simulink library "sm_solar_tracker_lib"  (R2021b)
settings: Solver=VariableStepAuto  StartTime=0.0  StopTime=10.0  RelTol=1e-3
undefined symbols (not defined in the file or in its folder): X, Y, Z
libraries: sm_lib x89, $bdroot x18
(part 1 of 3)
Description:
  | Solar Tracker Library
settings Model: Creator=The MathWorks, Inc.  LastModifiedBy=The MathWorks, Inc.
settings SolverCC: AlgebraicLoopSolver=TrustRegion
settings DataIOCC: ReturnWorkspaceOutputs=off
settings DebuggingCC: SFMachineParentedDataDiag=warning  ArithmeticOperatorsInVariantConditions=warning
settings SFSimCC: SimUseLocalCustomCode=off  CustomCodeUndefinedFunction=UseInterfaceOnly
settings RTWCC: RTWUseLocalCustomCode=off
settings CodeAppCC: StateflowObjectComments=on
settings ConfigComp: CovMetricSettings=dswe

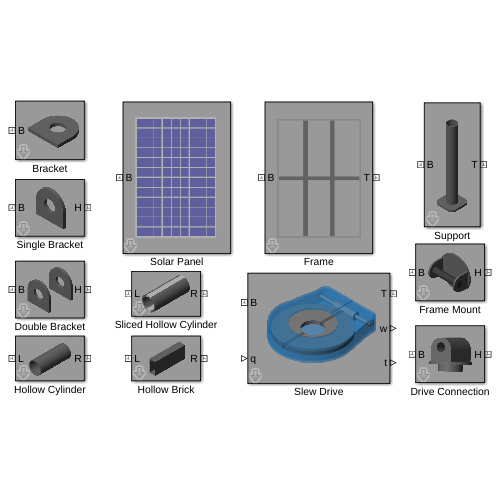
[thumbnail: Simulink's stored preview of the top-level diagram]
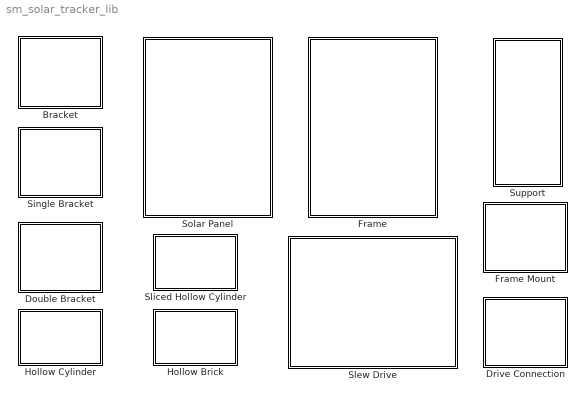
== system sm_solar_tracker_lib ==
  Bracket : Subsystem  mask(Bracket){height=0.1, width=0.1, thickness=0.01, holeOffset=0.05, holeRadius=0.02, rho=2700, color=[0.5 0.5 0.5]}
      mask prompts: height "Height (m)"; width "Width (m)"; thickness "Thickness (m)"; holeOffset "Hole Offset (m)"; holeRadius "Hole Radius (m)"; rho "Density (kg/m^3)"; color "Color [r g b]"
      mask help:
      | This block models a bracket element.
      |
      | Port B corresponds to the center point of the base face.
      mask init:
      | points = 40;
      | 
      | y = height - 0.5*width;
      | 
      | outerVertices = ...
      |   [          0      0;...
      |      0.5*width      0;...
      |      0.5*width      y;...
      |      0.5*width height;...
      |     -0.5*width height;...
      |     -0.5*width      y;...
      |     -0.5*width      0;...
      |              0      0];
      | 
      | outer = simmechanics.demohelpers.round_corners(...
      |   outerVertices, [4 5], 0.5*width, points);
      | 
      | holeTheta = linspace(1.5*pi, -0.5*pi, points);
      | 
      | hole = [holeRadius*cos(holeTheta);...
      |         holeRadius*sin(holeTheta)+holeOffset]';
      | 
      | crossSection = [hole; outer];
      mask DialogControl Tab1 Prompt: Dimensions
      mask DialogControl Tab2 Prompt: Material Properties
      mask Display:
      | image(fullfile(matlabroot,'toolbox','physmod','sm','smdemos','solar_tracker','images','sm_solar_tracker_bracket.png'));
      | port_label('lconn',1,'B');
  Double Bracket : Subsystem  mask(Double Bracket){height=0.75, width=0.75, thickness=0.15, offset=0.8, holeOffset=0.5, holeRadius=0.075, rho=7800, color=[0.3 0.3 0.3]}
      mask prompts: height "Height (m)"; width "Width (m)"; thickness "Thickness (m)"; offset "Offset (m)"; holeOffset "Hole Offset (m)"; holeRadius "Hole Radius (m)"; rho "Density (kg/m^3)"; color "Color [r g b]"
      mask help:
      | This block models a double bracket element.
      |
      | Port B corresponds to the midpoint between the base faces of the two elements. Port H corresponds to the midpoint between the two holes.
      mask DialogControl Tab1 Prompt: Dimensions
      mask DialogControl Tab2 Prompt: Material Properties
      mask Display:
      | image(fullfile(matlabroot,'toolbox','physmod','sm','smdemos','solar_tracker','images','sm_solar_tracker_double_bracket.png'));
      | port_label('lconn',1,'B');
      | port_label('rconn',1,'H');
  Drive Connection : Subsystem  mask(Drive Connection){connRadius=0.05, connThickness=0.005, connLength=0.03, bracketWidth=0.1, bracketThickness=0.15, holeRadius=0.02, holeOffset=0.06, baseThickness=0.01, rho=2700, color=[0.5 0.5 0.5]}
      mask prompts: connRadius "Connection Radius (m)"; connThickness "Connection Thickness (m)"; connLength "Connection Length (m)"; bracketWidth "Bracket Width and Height (m)"; bracketThickness "Bracket Thickness (m)"; holeRadius "Hole Radius (m)"; holeOffset "Hole Offset (m)"; baseThickness "Base Thickness (m)"; rho "Density (kg/m^3)"; color "Color [r g b]"
      mask help:
      | This block models the element that connects the solar array assembly to the slew drive.
      |
      | Port B corresponds to the center of the base face of the drive connection. Port H corresponds to the center of the bracket hole.
      mask init:
      | baseAngle = atan(bracketWidth / bracketThickness);
      | baseRadius = 0.5 * bracketThickness / cos(baseAngle);
      mask DialogControl Tab1 Prompt: Dimensions
      mask DialogControl Tab2 Prompt: Material Properties
      mask Display:
      | image(fullfile(matlabroot,'toolbox','physmod','sm','smdemos','solar_tracker','images','sm_solar_tracker_drive_connection.png'));
      | port_label('lconn',1,'B');
      | port_label('rconn',1,'H');
  Frame : Subsystem  mask(Frame){width=1, height=1.414, depth=0.1, beamWidth=0.05, beamThickness=0.01, frameWidth=0.02, frameThickness=0.005, rho=2700, beamColor=[0.5 0.5 0.5], frameColor=[0.7 0.7 0.7]}
      mask prompts: width "Width (m)"; height "Height (m)"; depth "Depth (m)"; beamWidth "Beam Width (m)"; beamThickness "Beam Thickness (m)"; frameWidth "Frame Width (m)"; frameThickness "Frame Thickness (m)"; rho "Density (kg/m^3)"; beamColor "Beam Color [r g b]"; frameColor "Frame Color [r g b]"
      mask help:
      | This block models the mounting frame of the solar tracker.
      |
      | Port B corresponds to the center of the base face of the horizontal beam. Port T corresponds to the center of the top face of the horizontal beam.
      mask init:
      | horizBeamLength = width - 2*frameWidth;
      | vertBeamLength = height - 2*frameWidth;
      | 
      | vertBeam1_offset = [-0.5*vertBeamLength 0 -(1/3)*horizBeamLength];
      | vertBeam2_offset = [-0.5*vertBeamLength 0 -(2/3)*horizBeamLength];
      | 
      | baseOffset = [0 -0.5*depth 0.5*horizBeamLength];
      | topOffset  = [0  0.5*depth 0.5*horizBeamLength];
      | 
      | leftFrameOffset  = [-0.5*height 0 -0.5*frameWidth];
      | rightFrameOffset = [-0.5*height 0  0.5*frameWidth];
      | 
      | nearFarFrameOffset = 0.5*height-0.5*frameWidth;
      mask DialogControl Tab1 Prompt: Dimensions
      mask DialogControl Tab2 Prompt: Material Properties
      mask Display:
      | image(fullfile(matlabroot,'toolbox','physmod','sm','smdemos','solar_tracker','images','sm_solar_tracker_frame.png'));
      | port_label('lconn',1,'B');
      | port_label('rconn',1,'T');
  Frame Mount : Subsystem  mask(Frame Mount){bracketWidth=0.1, bracketThickness=0.01, bracketOffset=0.18, holeRadius=0.02, holeOffset=0.06, baseThickness=0.01, rho=2700, mountColor=[0.5 0.5 0.5], pinColor=[0.3 0.3 0.3]}
      mask prompts: bracketWidth "Bracket Width and Height (m)"; bracketThickness "Bracket Thickness (m)"; bracketOffset "Bracket Offset (m)"; holeRadius "Hole Radius (m)"; holeOffset "Hole Offset (m)"; baseThickness "Base Thickness (m)"; rho "Density (kg/m^3)"; mountColor "Mount Color [r g b]"; pinColor "Pin Color [r g b]"
      mask help:
      | This block models the mount for the frame of the solar tracker.
      |
      | Port B corresponds to the center of the base plate. Port H corresponds to the center point of the pin that passes through the holes of the bracket.
      mask init:
      | baseAngle = atan(bracketWidth / (bracketOffset + bracketThickness));
      | baseRadius = 0.5*bracketWidth / sin(baseAngle);
      | pinLength = bracketOffset + bracketThickness;
      mask DialogControl Tab1 Prompt: Dimensions
      mask DialogControl Tab2 Prompt: Material Properties
      mask Display:
      | image(fullfile(matlabroot,'toolbox','physmod','sm','smdemos','solar_tracker','images','sm_solar_tracker_frame_mount.png'));
      | port_label('lconn',1,'B');
      | port_label('rconn',1,'H');
  Hollow Brick : Subsystem  mask(Hollow Brick){width=0.1, depth=0.2, length=0.5, thickness=0.01, rho=2700, color=[0.5 0.5 0.5]}
      mask prompts: width "Width (m)"; depth "Depth (m)"; length "Length (m)"; thickness "Thickness (m)"; rho "Density (kg/m^3)"; color "Color [r g b]"
      mask help:
      | This block models a hollow brick element.
      |
      | Port L corresponds to the left-hand end of the brick. Port R corresponds to the right-hand end of the brick.
      mask init:
      | halfWidth = 0.5*width;
      | halfDepth = 0.5*depth;
      | 
      | halfInnerWidth = 0.5*(width - 2*thickness);
      | halfInnerDepth = 0.5*(depth - 2*thickness);
      | 
      | crossSection = [...
      |   -halfInnerWidth -halfInnerDepth;...
      |   -halfInnerWidth  halfInnerDepth;...
      |    halfInnerWidth  halfInnerDepth;...
      |    halfInnerWidth -halfInnerDepth;...
      |   -halfInnerWidth -halfInnerDepth;...
      |   -halfWidth      -halfDepth;...
      |    halfWidth      -halfDepth;...
      |    halfWidth       halfDepth;...
      |   -halfWidth       halfDepth;...
      |   -halfWidth      -halfDepth];
      mask DialogControl Tab1 Prompt: Dimensions
      mask DialogControl Tab2 Prompt: Material Properties
      mask Display:
      | image(fullfile(matlabroot,'toolbox','physmod','sm','smdemos','solar_tracker','images','sm_solar_tracker_hollow_brick.png'));
      | port_label('lconn',1,'L');
      | port_label('rconn',1,'R');
  Hollow Cylinder : Subsystem  mask(Hollow Cylinder){outerRadius=0.1, thickness=0.01, length=0.5, rho=2700, color=[0.5 0.5 0.5]}
      mask prompts: outerRadius "Outer Radius (m)"; thickness "Thickness (m)"; length "Length (m)"; rho "Density (kg/m^3)"; color "Color [r g b]"
      mask help:
      | This block models a hollow cylinder element.
      |
      | Port L corresponds to the left-hand end of the cylinder. Port R corresponds to the right-hand end of the cylinder.
      mask init:
      | innerRadius = outerRadius - thickness;
      | 
      | halfLength = 0.5*length;
      | 
      | crossSection = [...
      |   innerRadius -halfLength;...
      |   outerRadius -halfLength;...
      |   outerRadius  halfLength;...
      |   innerRadius  halfLength];
      mask DialogControl Tab1 Prompt: Dimensions
      mask DialogControl Tab2 Prompt: Material Properties
      mask Display:
      | image(fullfile(matlabroot,'toolbox','physmod','sm','smdemos','solar_tracker','images','sm_solar_tracker_hollow_cylinder.png'));
      | port_label('lconn',1,'L');
      | port_label('rconn',1,'R');
  Single Bracket : Subsystem  mask(Single Bracket){height=0.1, width=0.1, thickness=0.01, holeOffset=0.05, holeRadius=0.02, rho=2700, color=[0.5 0.5 0.5]}
      mask prompts: height "Height (m)"; width "Width (m)"; thickness "Thickness (m)"; holeOffset "Hole Offset (m)"; holeRadius "Hole Radius (m)"; rho "Density (kg/m^3)"; color "Color [r g b]"
      mask help:
      | This block models a bracket element.
      |
      | Port B corresponds to the center point of the base face. Port H corresponds to the center of the hole.
      mask DialogControl Tab1 Prompt: Dimensions
      mask DialogControl Tab2 Prompt: Material Properties
      mask Display:
      | image(fullfile(matlabroot,'toolbox','physmod','sm','smdemos','solar_tracker','images','sm_solar_tracker_single_bracket.png'));
      | port_label('lconn',1,'B');
      | port_label('rconn',1,'H');
  Slew Drive : Subsystem  mask(Slew Drive){wormLeadAngle=10, wormLength=0.17, gearOuterRadius=0.1, gearInnerRadius=0.03, gearExposedRadius=0.06, ratio=50, housingThickness=0.005, bWormRevolute=1e-6, wormRho=7800, gearRho=7800, housingRho=2700, wormColor=[0.7 0.7 0.7], gearColor=[0.6 0.6 0.6], housingColor=[0.1 0.6 1.0], housingOpacity=0.3}
      mask prompts: wormLeadAngle "Worm Lead Angle (deg)"; wormLength "Worm Length (m)"; gearOuterRadius "Gear Outer Radius (m)"; gearInnerRadius "Gear Inner Radius (m)"; gearExposedRadius "Gear Exposed Radius (m)"; ratio "Ratio (Ng / Nw)"; housingThickness "Housing Thickness (m)"; bWormRevolute "Worm Revolute Damping (Nm/(deg/s))"; wormRho "Worm Density (kg/m^3)"; gearRho "Gear Density (kg/m^3)"; housingRho "Housing Density (kg/m3)"; wormColor "Worm Color [r g b]"; gearColor "Gear Color [r g b]"; housingColor "Housing Color [r g b]"; housingOpacity "Housing Opacity"
      mask help:
      | This block models the slew drive of the solar tracker.
      |
      | Port B corresponds to the base face of the housing aligned with the gear axis. Port T corresponds to the center of the top face of the gear.
      |
      | Input port q specifies the motion actuation signal of the gear revolute. Output port w corresponds to the angular velocity of the worm revolute. Output port t corresponds to the automatically computed actuation torque at the worm revolute necessary to achieve the desired motion signal of the gear revolute.
      mask init:
      | % Worm Properties
      | wormRadius            = gearOuterRadius / (ratio * tand(wormLeadAngle));
      | wormNonThreadedRadius = 0.4*wormRadius;
      | 
      | wormThreadedLength    = 0.4*wormLength;
      | wormNonThreadedLength = 0.5*(wormLength - wormThreadedLength);
      | 
      | wormHoleRadius = 0.5*wormNonThreadedRadius;
      | 
      | wormThreadedThickness    = wormRadius - wormHoleRadius;
      | wormNonThreadedThickness = wormNonThreadedRadius - wormHoleRadius;
      | 
      | wormSliceColor      = 0.75*wormColor;
      | wormSliceProportion = 0.25;
      | 
      | % Worm Offsets
      | wormLeftOffset  = [-0.5*wormLength gearOuterRadius+wormRadius 0];
      | wormRightOffset = [ 0.5*wormLength gearOuterRadius+wormRadius 0];
      | 
      | % Gear Properties
      | gearLength         = wormRadius;
      | gearThickness      = gearOuterRadius - gearInnerRadius;
      | gearSliceThickness = 0.1*gearOuterRadius;
      | gearSliceColor     = 0.75*gearColor;
      | 
      | % Housing Dimensions
      | housingRadTol = 0.05*gearOuterRadius;
      | sideDepth     = 2*wormRadius + 2*housingRadTol;
      | 
      | % Housing Base Vertices
      | baseVertex1_x = 0;
      | baseVertex2_x = housingThickness + housingRadTol + 2*wormRadius;
      | baseVertex3_x = baseVertex2_x + gearOuterRadius;
      | baseVertex4_x = baseVertex3_x + gearOuterRadius + housingRadTol + housingThickness;
      | 
      | baseVertex1_y = -0.5*wormLength - housingThickness;
      | baseVertex2_y = baseVertex1_y;
      | baseVertex3_y = -gearOuterRadius - housingRadTol - housingThickness;
      | baseVertex4_y = baseVertex3_y;
      | 
      | baseVertices = [...
      |   baseVertex1_x  baseVertex1_y;...
      |   baseVertex2_x  baseVertex2_y;...
      |   baseVertex3_x  baseVertex3_y;...
      |   baseVertex4_x  baseVertex4_y;...
      |   baseVertex4_x -baseVertex4_y;...
      |   baseVertex3_x -baseVertex3_y;...
      |   baseVertex2_x -baseVertex2_y;...
      |   baseVertex1_x -baseVertex1_y];
      | 
      | baseVertex1_R = 0.5*wormRadius + housingRadTol + housingThickness;
      | baseVertex4_R = gearOuterRadius + housingRadTol + housingThickness;
      | baseVertex5_R = baseVertex4_R;
      | baseVertex8_R = baseVertex1_R;
      | 
      | baseVerticesR = [baseVertex1_R baseVertex4_R baseVertex5_R baseVertex8_R];
      |   
      | baseVertices = simmechanics.demohelpers.round_corners(...
      |   baseVertices, [1 4 5 8], baseVerticesR, 20);
      | 
      | % Housing Side Vertices
      | sideVertices = [...
      |   baseVertex1_x+housingThickness  baseVertex1_y+housingThickness;...
      |   baseVertex2_x                   baseVertex2_y+housingThickness;...
      |   baseVertex3_x                   baseVertex3_y+housingThickness;...
      |   baseVertex4_x-housingThickness  baseVertex4_y+housingThickness;...
      |   baseVertex4_x-housingThickness -baseVertex4_y-housingThickness;...
      |   baseVertex3_x                  -baseVertex3_y-housingThickness;...
      |   baseVertex2_x                  -baseVertex2_y-housingThickness;...
      |   baseVertex1_x+housingThickness -baseVertex1_y-housingThickness];
      | 
      | sideVertex1_R = 0.5*wormRadius + housingRadTol;
      | sideVertex4_R = gearOuterRadius + housingRadTol;
      | sideVertex5_R = sideVertex4_R;
      | sideVertex8_R = sideVertex1_R;
      | 
      | sideVerticesR = [sideVertex1_R sideVertex4_R sideVertex5_R sideVertex8_R];
      | 
      | sideVertices = simmechanics.demohelpers.round_corners(...
      |   sideVertices, [1 4 5 8], sideVerticesR, 20);
      | 
      | sideVertices = flipud(sideVertices);
      | sideVertices(end+1,:) = sideVertices(1,:);
      | 
      | sideVertices = [sideVertices; baseVertices(end,:); baseVertices];
      | 
      | % Housing Top Vertices
      | topHoleOffset = housingThickness + housingRadTol + 2*wormRadius + gearOuterRadius;
      | 
      | topHoleTheta = linspace(pi, -pi, 40);
      | topVertices = [gearExposedRadius*cos(topHoleTheta)+topHoleOffset;...
      |                gearExposedRadius*sin(topHoleTheta)]';
      | 
      | topVertices = [topVertices; 0 0; baseVertices; 0 0];
      | 
      | % Housing Offsets
      | housingOffset        = topHoleOffset;
      | housingTopBaseOffset = 0.5*sideDepth + 0.5*housingThickness;
      | baseOffset           = [topHoleOffset 0 -0.5*housingThickness];
      mask DialogControl Tab1 Prompt: Dimensions
      mask DialogControl Tab2 Prompt: Internal Mechanics
      mask DialogControl Tab3 Prompt: Material Properties
      mask Display:
      | image(fullfile(matlabroot,'toolbox','physmod','sm','smdemos','solar_tracker','images','sm_solar_tracker_slew_drive.png'));
      | port_label('lconn',1,'B');
      | port_label('lconn',2,'q');
      | port_label('rconn',1,'T');
      | port_label('rconn',2,'w');
      | port_label('rconn',3,'t');
  Sliced Hollow Cylinder : Subsystem  mask(Sliced Hollow Cylinder){outerRadius=0.1, thickness=0.01, length=0.5, sliceThickness=0.02, rho=2700, mainColor=[0.5 0.5 0.5], sliceColor=[0.9 0.9 0.9]}
      mask prompts: outerRadius "Outer Radius (m)"; thickness "Thickness (m)"; length "Length (m)"; sliceThickness "Slice Thickness (m)"; rho "Density (kg/m^3)"; mainColor "Main Color [r g b]"; sliceColor "Slice Color [r g b]"
      mask help:
      | This block models a hollow cylinder where a slice of the cylinder can be set to a different color.
      |
      | Port L corresponds to the left-hand end of the cylinder. Port R corresponds to the right-hand end of the cylinder.
      mask init:
      | points = 30;
      | 
      | innerRadius = outerRadius - thickness;
      | 
      | outerTheta = acos(0.5*sliceThickness / outerRadius);
      | 
      | rightOuterThetaVect = linspace(  -outerTheta,      outerTheta, points);
      | leftOuterThetaVect  = linspace(pi-outerTheta,   pi+outerTheta, points);
      | topOuterThetaVect   = linspace(   outerTheta,   pi-outerTheta, points);
      | botOuterThetaVect   = linspace(pi+outerTheta, 2*pi-outerTheta, points);
      | 
      | if (sliceThickness > 2*innerRadius)
      |   % The slice is wider than the hole
      |   rightCrossSection = [outerRadius*cos(rightOuterThetaVect);...
      |                        outerRadius*sin(rightOuterThetaVect)]';
      |   leftCrossSection  = [outerRadius*cos(leftOuterThetaVect);...
      |                        outerRadius*sin(leftOuterThetaVect)]';
      | 
      |   topInnerThetaVect = linspace(pi, 0, points);
      |   botInnerThetaVect = linspace(0, -pi, points);
      |   
      |   topCrossSection = [...
      |     outerRadius*cos(topOuterThetaVect) -0.5*sliceThickness innerRadius*cos(topInnerThetaVect) 0.5*sliceThickness;...
      |     outerRadius*sin(topOuterThetaVect) 0 innerRadius*sin(topInnerThetaVect) 0]';
      |   
      |   botCrossSection = [...
      |     outerRadius*cos(botOuterThetaVect) 0.5*sliceThickness innerRadius*cos(botInnerThetaVect) -0.5*sliceThickness;...
      |     outerRadius*sin(botOuterThetaVect) 0 innerRadius*sin(botInnerThetaVect) 0]';
      | else
      |   % The slicer is narrower than the hole
      |   innerTheta = acos(0.5*sliceThickness / innerRadius);
      |   
      |   rightInnerThetaVect = linspace(   innerTheta,    -innerTheta, points);
      |   leftInnerThetaVect  = linspace(pi+innerTheta,  pi-innerTheta, points);
      |   topInnerThetaVect   = linspace(pi-innerTheta,     innerTheta, points);
      |   botInnerThetaVect   = linspace(  -innerTheta, -pi+innerTheta, points);
      |   
      |   rightCrossSection = [...
      |     outerRadius*cos(rightOuterThetaVect) innerRadius*cos(rightInnerThetaVect);...
      |     outerRadius*sin(rightOuterThetaVect) innerRadius*sin(rightInnerThetaVect)]';
      |   leftCrossSection  = [...
      |     outerRadius*cos(leftOuterThetaVect)  innerRadius*cos(leftInnerThetaVect);...
      |     outerRadius*sin(leftOuterThetaVect)  innerRadius*sin(leftInnerThetaVect)]';
      |   topCrossSection   = [...
      |     outerRadius*cos(topOuterThetaVect)   innerRadius*cos(topInnerThetaVect);...
      |     outerRadius*sin(topOuterThetaVect)   innerRadius*sin(topInnerThetaVect)]';
      |   botCrossSection   = [...
      |     outerRadius*cos(botOuterThetaVect)   innerRadius*cos(botInnerThetaVect);...
      |     outerRadius*sin(botOuterThetaVect)   innerRadius*sin(botInnerThetaVect)]';
      | end
      mask DialogControl Tab1 Prompt: Dimensions
      mask DialogControl Tab2 Prompt: Material Properties
      mask Display:
      | image(fullfile(matlabroot,'toolbox','physmod','sm','smdemos','solar_tracker','images','sm_solar_tracker_sliced_hollow_cylinder.png'));
      | port_label('lconn',1,'L');
      | port_label('rconn',1,'R');
  Solar Panel : Subsystem  mask(Solar Panel){width=1, height=1.414, frameWidth=0.02, frameDepth=0.01, cellsRho=100, frameRho=950, cellsColor=[0 0 0.5], frameColor=[0.9 0.9 0.9]}
      mask prompts: width "Width (m)"; height "Height (m)"; frameWidth "Frame Width (m)"; frameDepth "Frame Depth (m)"; cellsRho "Cell Density (kg/m^3)"; frameRho "Frame Density (kg/m^3)"; cellsColor "Cell Color [r g b]"; frameColor "Frame Color [r g b]"
      mask help:
      | This block models the solar panel of the solar tracker.
      |
      | Port B corresponds to the center of the base face.
      mask init:
      | % Solar cells
      | cellsDim = ...
      |   [width-2*frameWidth, height-2*frameWidth, 0.25*frameDepth];
      | 
      | % Frame base and edges
      | frameBaseDim = [width height 0.25*frameDepth];
      | frameVertEdgeDim = [frameWidth height 0.75*frameDepth];
      | frameHorizEdgeDim = [width-2*frameWidth frameWidth 0.75*frameDepth];
      | 
      | % Horizontal dividers
      | frameMajorHorizDim = frameHorizEdgeDim;
      | frameMinorHorizDim = ...
      |   [width-2*frameWidth 0.5*frameWidth 0.25*frameDepth];
      | 
      | frameMinorHorizSpacing = (1/12)*(height-frameWidth);
      | frameMinorHorizOffsetZ = -0.25*frameDepth;
      | 
      | frameMinorHoriz1_offset  = ...
      |   [0  5*frameMinorHorizSpacing frameMinorHorizOffsetZ];
      | frameMinorHoriz2_offset  = ...
      |   [0  4*frameMinorHorizSpacing frameMinorHorizOffsetZ];
      | frameMinorHoriz3_offset  = ...
      |   [0  3*frameMinorHorizSpacing frameMinorHorizOffsetZ];
      | frameMinorHoriz4_offset  = ...
      |   [0  2*frameMinorHorizSpacing frameMinorHorizOffsetZ];
      | frameMinorHoriz5_offset  = ...
      |   [0  1*frameMinorHorizSpacing frameMinorHorizOffsetZ];
      | frameMinorHoriz6_offset  = ...
      |   [0 -1*frameMinorHorizSpacing frameMinorHorizOffsetZ];
      | frameMinorHoriz7_offset  = ...
      |   [0 -2*frameMinorHorizSpacing frameMinorHorizOffsetZ];
      | frameMinorHoriz8_offset  = ...
      |   [0 -3*frameMinorHorizSpacing frameMinorHorizOffsetZ];
      | frameMinorHoriz9_offset  = ...
      |   [0 -4*frameMinorHorizSpacing frameMinorHorizOffsetZ];
      | frameMinorHoriz10_offset = ...
      |   [0 -5*frameMinorHorizSpacing frameMinorHorizOffsetZ];
      | 
      | % Vertical dividers
      | frameMajorVertDim = ...
      |   [frameWidth height-2*frameWidth 0.5*frameDepth];
      | frameMinorVertDim = ...
      |   [0.25*frameWidth height-2*frameWidth 0.125*frameDepth];
      | 
      | frameMajorVertOffset = (1/6)*width;
      | frameMinorVertSpacing = (1/18)*(width-frameWidth);
      | frameMinorVertOffsetZ = -(0.5*frameDepth-frameMinorVertDim(3));
      | 
      | frameMinorVert1_offset = ...
      |   [-7*frameMinorVertSpacing 0 frameMinorVertOffsetZ];
      | frameMinorVert2_offset = ...
      |   [-5*frameMinorVertSpacing 0 frameMinorVertOffsetZ];
      | frameMinorVert3_offset = ...
      |   [-1*frameMinorVertSpacing 0 frameMinorVertOffsetZ];
      | frameMinorVert4_offset = ...
      |   [ 1*frameMinorVertSpacing 0 frameMinorVertOffsetZ];
      | frameMinorVert5_offset = ...
      |   [ 5*frameMinorVertSpacing 0 frameMinorVertOffsetZ];
      | frameMinorVert6_offset = ...
      |   [ 7*frameMinorVertSpacing 0 frameMinorVertOffsetZ];
      mask DialogControl Tab1 Prompt: Dimensions
      mask DialogControl Tab2 Prompt: Material Properties
      mask Display:
      | image(fullfile(matlabroot,'toolbox','physmod','sm','smdemos','solar_tracker','images','sm_solar_tracker_solar_panel.png'));
      | port_label('lconn',1,'B');
  Support : Subsystem  mask(Support){columnRadius=0.05, columnThickness=0.005, columnHeight=0.9, baseWidth=0.2, baseThickness=0.02, rho=2700, color=[0.5 0.5 0.5]}
      mask prompts: columnRadius "Column Radius (m)"; columnThickness "Column Thickness (m)"; columnHeight "Column Height (m)"; baseWidth "Base Width (m)"; baseThickness "Base Thickness (m)"; rho "Density (kg/m^3)"; color "Color [r g b]"
      mask help:
      | This block models the support for the solar tracker.
      |
      | Port B corresponds to the center of the base face. Port T corresponds to the center of the top face of the column.
      mask init:
      | halfBaseWidth = 0.5*baseWidth;
      | 
      | baseVertices = [...
      |   -halfBaseWidth -halfBaseWidth;...
      |    halfBaseWidth -halfBaseWidth;...
      |    halfBaseWidth  halfBaseWidth;...
      |   -halfBaseWidth  halfBaseWidth];
      | 
      | baseVertices = simmechanics.demohelpers.round_corners(...
      |   baseVertices, [1:4], 0.5*halfBaseWidth, 10);
      mask DialogControl Tab1 Prompt: Dimensions
      mask DialogControl Tab2 Prompt: Material Properties
      mask Display:
      | image(fullfile(matlabroot,'toolbox','physmod','sm','smdemos','solar_tracker','images','sm_solar_tracker_support.png'));
      | port_label('lconn',1,'B');
      | port_label('rconn',1,'T');

== system sm_solar_tracker_lib/Bracket ==
  Bracket : sm_lib/Body Elements/Extruded Solid  GraphicAmbientColor=[0.15 0.15 0.15 1.0]  BasedOnType=Density  CenterOfMass=[0 0 0]  CenterOfMassUnits=m  GraphicDiffuseColor=color  ExportConvexHullGeometry=off  ExtrusionCrossSection=crossSection  ExtrusionCrossSectionUnits=m  Density=rho  DensityUnits=kg/m^3  DoExposeReferenceFrame=on  GraphicEmissiveColor=[0.0 0.0 0.0 1.0]  ExportEntireGeometry=off  ExtrusionLength=thickness  ExtrusionLengthUnits=m  ExtrusionType=General  SerializedFrames=<Frames/>  MarkerShape=Sphere  MarkerSize=10  GraphicType=FromGeometry  InertiaType=CalculateFromGeometry  Mass=1  MassUnits=kg  MomentsOfInertia=[1 1 1]  MomentsOfInertiaUnits=kg*m^2  PolygonNumSides=3  GraphicOpacity=1.0  PolygonOuterRadius=1  PolygonOuterRadiusUnits=m  ProductsOfInertia=[1 1 1]  ProductsOfInertiaUnits=kg*m^2  GraphicShininess=75  GraphicSpecularColor=[0.5 0.5 0.5 1.0]  GraphicVisPropType=SimpleVisualProperties
  B : PMIOPort  Side=Left
  connections:
  Bracket/RConn1 -- B/RConn1

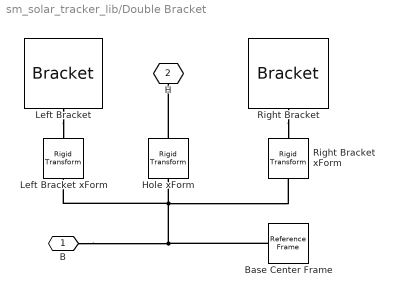
== system sm_solar_tracker_lib/Double Bracket ==
  Base Center Frame : sm_lib/Frames and Transforms/Reference Frame
  Hole xForm : sm_lib/Frames and Transforms/Rigid Transform  TranslationMethod=StandardAxis  TranslationStandardOffset=holeOffset  TranslationLengthUnit=m  TranslationStandardAxis=+Z  TranslationCartesianOffset=[0 0 0]  TranslationROffset=0  TranslationROffsetUnits=m  TranslationZOffset=0  TranslationZOffsetUnits=m  TranslationThetaOffset=0  TranslationThetaOffsetUnits=deg  RotationMethod=AlignedAxes  RotationAngleUnits=deg  RotationStandardAxis=+X  RotationAngle=90  RotationArbitraryAxis=[0 0 1]  FollAlignAxisA=+X  BaseAlignAxisA=+X  FollAlignAxisB=+Y  BaseAlignAxisB=+Z  RotationSequenceAxes=FollowerAxes  RotationSequence=XYX  RotationSequenceAngles=[0 0 0]  RotationSequenceAnglesUnits=deg  RotationMatrix=[1 0 0; 0 1 0; 0 0 1]
  Left Bracket : $bdroot/Bracket  height=height  width=width  thickness=thickness  holeOffset=holeOffset  holeRadius=holeRadius  rho=rho  color=color
  Left Bracket xForm : sm_lib/Frames and Transforms/Rigid Transform  TranslationMethod=StandardAxis  TranslationStandardOffset=0.5*offset  TranslationLengthUnit=m  TranslationStandardAxis=-Y  TranslationCartesianOffset=[0 0 0]  TranslationROffset=0  TranslationROffsetUnits=m  TranslationZOffset=0  TranslationZOffsetUnits=m  TranslationThetaOffset=0  TranslationThetaOffsetUnits=deg  RotationMethod=AlignedAxes  RotationAngleUnits=deg  RotationStandardAxis=+X  RotationAngle=90  RotationArbitraryAxis=[0 0 1]  FollAlignAxisA=+X  BaseAlignAxisA=+X  FollAlignAxisB=+Y  BaseAlignAxisB=+Z  RotationSequenceAxes=FollowerAxes  RotationSequence=XYX  RotationSequenceAngles=[0 0 0]  RotationSequenceAnglesUnits=deg  RotationMatrix=[1 0 0; 0 1 0; 0 0 1]
  Right Bracket : $bdroot/Bracket  height=height  width=width  thickness=thickness  holeOffset=holeOffset  holeRadius=holeRadius  rho=rho  color=color
  Right Bracket xForm : sm_lib/Frames and Transforms/Rigid Transform  TranslationMethod=StandardAxis  TranslationStandardOffset=0.5*offset  TranslationLengthUnit=m  TranslationStandardAxis=+Y  TranslationCartesianOffset=[0 0 0]  TranslationROffset=0  TranslationROffsetUnits=m  TranslationZOffset=0  TranslationZOffsetUnits=m  TranslationThetaOffset=0  TranslationThetaOffsetUnits=deg  RotationMethod=AlignedAxes  RotationAngleUnits=deg  RotationStandardAxis=+X  RotationAngle=90  RotationArbitraryAxis=[0 0 1]  FollAlignAxisA=+X  BaseAlignAxisA=+X  FollAlignAxisB=+Y  BaseAlignAxisB=+Z  RotationSequenceAxes=FollowerAxes  RotationSequence=XYX  RotationSequenceAngles=[0 0 0]  RotationSequenceAnglesUnits=deg  RotationMatrix=[1 0 0; 0 1 0; 0 0 1]
  B : PMIOPort  Side=Left
  H : PMIOPort  Port=2  Side=Right
  connections:
  Hole xForm/LConn1 -- B/RConn1 -- Base Center Frame/RConn1 -- Right Bracket xForm/LConn1 -- Left Bracket xForm/LConn1
  Right Bracket/LConn1 -- Right Bracket xForm/RConn1
  Hole xForm/RConn1 -- H/RConn1
  Left Bracket/LConn1 -- Left Bracket xForm/RConn1

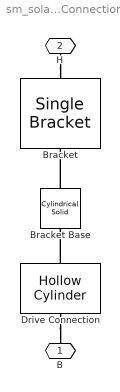
== system sm_solar_tracker_lib/Drive Connection ==
  Bracket : $bdroot/Single Bracket  height=bracketWidth  width=bracketWidth  thickness=bracketThickness  holeOffset=holeOffset  holeRadius=holeRadius  rho=rho  color=color
  Bracket Base : sm_lib/Body Elements/Cylindrical Solid  GraphicAmbientColor=[0.15 0.15 0.15 1.0]  BasedOnType=Density  CenterOfMass=[0 0 0]  CenterOfMassUnits=m  GraphicDiffuseColor=color  CylinderLength=baseThickness  CylinderLengthUnits=m  CylinderRadius=baseRadius  CylinderRadiusUnits=m  Density=rho  DensityUnits=kg/m^3  DoExposeReferenceFrame=off  GraphicEmissiveColor=[0.0 0.0 0.0 1.0]  ExportEntireGeometry=off  SerializedFrames=<Frames><Frame><Id>Frame1</Id><Value><Name>T</Name><Origin><Source>GeometricFeature</Source><FeatureName>top surface</FeatureName></Origin><PrimaryAxis><DefinedDirection>+Z</DefinedDirection><Source>ReferenceFrame</Source><SourceDirection>+Z</SourceDirection><FeatureName></FeatureName></PrimaryAxis><SecondaryAxis><DefinedDirection>+X</DefinedDirection><Source>ReferenceFrame</Source><SourceDirection>-Y</SourceDirection><FeatureName></FeatureName></SecondaryAxis></Value></Frame><Frame><Id>Frame2</Id><Value><Name>B</Name><Origin><Source>GeometricFeature</Source><FeatureName>bottom surface</FeatureName></Origin><PrimaryAxis><DefinedDirection>+Z</DefinedDirection><Source>ReferenceFrame</Source><SourceDirection>+Z</SourceDirection><FeatureName></FeatureName></PrimaryAxis><SecondaryAxis><DefinedDirection>+X</DefinedDirection><Source>ReferenceFrame</Source><SourceDirection>+X</SourceDirection><FeatureName></FeatureName></SecondaryAxis></Value></Frame></Frames>  MarkerShape=Sphere  MarkerSize=10  GraphicType=FromGeometry  InertiaType=CalculateFromGeometry  Mass=1  MassUnits=kg  MomentsOfInertia=[1 1 1]  MomentsOfInertiaUnits=kg*m^2  GraphicOpacity=1.0  ProductsOfInertia=[1 1 1]  ProductsOfInertiaUnits=kg*m^2  GraphicShininess=75  GraphicSpecularColor=[0.5 0.5 0.5 1.0]  GraphicVisPropType=SimpleVisualProperties
  Drive Connection : $bdroot/Hollow Cylinder  outerRadius=connRadius  thickness=connThickness  length=connLength  rho=rho  color=color
  B : PMIOPort  Side=Left
  H : PMIOPort  Port=2  Side=Right
  connections:
  H/RConn1 -- Bracket/RConn1
  Bracket Base/LConn1 -- Bracket/LConn1
  Drive Connection/RConn1 -- Bracket Base/RConn1
  Drive Connection/LConn1 -- B/RConn1

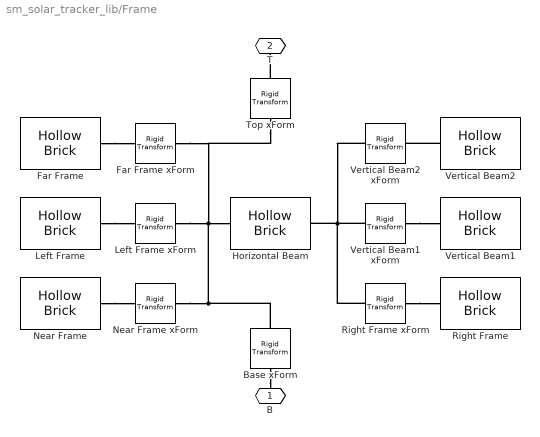
== system sm_solar_tracker_lib/Frame ==
  Base xForm : sm_lib/Frames and Transforms/Rigid Transform  TranslationMethod=Cartesian  TranslationStandardOffset=0  TranslationLengthUnit=m  TranslationStandardAxis=+Z  TranslationCartesianOffset=baseOffset  TranslationROffset=0  TranslationROffsetUnits=m  TranslationZOffset=0  TranslationZOffsetUnits=m  TranslationThetaOffset=0  TranslationThetaOffsetUnits=deg  RotationMethod=AlignedAxes  RotationAngleUnits=deg  RotationStandardAxis=+Z  RotationAngle=0.0  RotationArbitraryAxis=[0 0 1]  FollAlignAxisA=+Z  BaseAlignAxisA=+Y  FollAlignAxisB=+X  BaseAlignAxisB=+Z  RotationSequenceAxes=FollowerAxes  RotationSequence=XYX  RotationSequenceAngles=[0 0 0]  RotationSequenceAnglesUnits=deg  RotationMatrix=[1 0 0; 0 1 0; 0 0 1]
  Far Frame : $bdroot/Hollow Brick  width=frameWidth  depth=depth  length=horizBeamLength  thickness=frameThickness  rho=rho  color=frameColor
  Far Frame xForm : sm_lib/Frames and Transforms/Rigid Transform  TranslationMethod=StandardAxis  TranslationStandardOffset=nearFarFrameOffset  TranslationLengthUnit=m  TranslationStandardAxis=+X  TranslationCartesianOffset=[0 0 0]  TranslationROffset=0  TranslationROffsetUnits=m  TranslationZOffset=0  TranslationZOffsetUnits=m  TranslationThetaOffset=0  TranslationThetaOffsetUnits=deg  RotationMethod=None  RotationAngleUnits=deg  RotationStandardAxis=+Z  RotationAngle=0.0  RotationArbitraryAxis=[0 0 1]  FollAlignAxisA=+X  BaseAlignAxisA=+Y  FollAlignAxisB=+Y  BaseAlignAxisB=+Z  RotationSequenceAxes=FollowerAxes  RotationSequence=XYX  RotationSequenceAngles=[0 0 0]  RotationSequenceAnglesUnits=deg  RotationMatrix=[1 0 0; 0 1 0; 0 0 1]
  Horizontal Beam : $bdroot/Hollow Brick  width=beamWidth  depth=depth  length=horizBeamLength  thickness=beamThickness  rho=rho  color=beamColor
  Left Frame : $bdroot/Hollow Brick  width=frameWidth  depth=depth  length=height  thickness=frameThickness  rho=rho  color=frameColor
  Left Frame xForm : sm_lib/Frames and Transforms/Rigid Transform  TranslationMethod=Cartesian  TranslationStandardOffset=0  TranslationLengthUnit=m  TranslationStandardAxis=+Z  TranslationCartesianOffset=leftFrameOffset  TranslationROffset=0  TranslationROffsetUnits=m  TranslationZOffset=0  TranslationZOffsetUnits=m  TranslationThetaOffset=0  TranslationThetaOffsetUnits=deg  RotationMethod=AlignedAxes  RotationAngleUnits=deg  RotationStandardAxis=+Z  RotationAngle=0.0  RotationArbitraryAxis=[0 0 1]  FollAlignAxisA=+Z  BaseAlignAxisA=+X  FollAlignAxisB=+X  BaseAlignAxisB=+Z  RotationSequenceAxes=FollowerAxes  RotationSequence=XYX  RotationSequenceAngles=[0 0 0]  RotationSequenceAnglesUnits=deg  RotationMatrix=[1 0 0; 0 1 0; 0 0 1]
  Near Frame : $bdroot/Hollow Brick  width=frameWidth  depth=depth  length=horizBeamLength  thickness=frameThickness  rho=rho  color=frameColor
  Near Frame xForm : sm_lib/Frames and Transforms/Rigid Transform  TranslationMethod=StandardAxis  TranslationStandardOffset=nearFarFrameOffset  TranslationLengthUnit=m  TranslationStandardAxis=-X  TranslationCartesianOffset=[0 0 0]  TranslationROffset=0  TranslationROffsetUnits=m  TranslationZOffset=0  TranslationZOffsetUnits=m  TranslationThetaOffset=0  TranslationThetaOffsetUnits=deg  RotationMethod=None  RotationAngleUnits=deg  RotationStandardAxis=+Z  RotationAngle=0.0  RotationArbitraryAxis=[0 0 1]  FollAlignAxisA=+X  BaseAlignAxisA=+Y  FollAlignAxisB=+Y  BaseAlignAxisB=+Z  RotationSequenceAxes=FollowerAxes  RotationSequence=XYX  RotationSequenceAngles=[0 0 0]  RotationSequenceAnglesUnits=deg  RotationMatrix=[1 0 0; 0 1 0; 0 0 1]
  Right Frame : $bdroot/Hollow Brick  width=frameWidth  depth=depth  length=height  thickness=frameThickness  rho=rho  color=frameColor
  Right Frame xForm : sm_lib/Frames and Transforms/Rigid Transform  TranslationMethod=Cartesian  TranslationStandardOffset=0  TranslationLengthUnit=m  TranslationStandardAxis=+Z  TranslationCartesianOffset=rightFrameOffset  TranslationROffset=0  TranslationROffsetUnits=m  TranslationZOffset=0  TranslationZOffsetUnits=m  TranslationThetaOffset=0  TranslationThetaOffsetUnits=deg  RotationMethod=AlignedAxes  RotationAngleUnits=deg  RotationStandardAxis=+Z  RotationAngle=0.0  RotationArbitraryAxis=[0 0 1]  FollAlignAxisA=+Z  BaseAlignAxisA=+X  FollAlignAxisB=+X  BaseAlignAxisB=+Z  RotationSequenceAxes=FollowerAxes  RotationSequence=XYX  RotationSequenceAngles=[0 0 0]  RotationSequenceAnglesUnits=deg  RotationMatrix=[1 0 0; 0 1 0; 0 0 1]
  Top xForm : sm_lib/Frames and Transforms/Rigid Transform  TranslationMethod=Cartesian  TranslationStandardOffset=0  TranslationLengthUnit=m  TranslationStandardAxis=+Z  TranslationCartesianOffset=topOffset  TranslationROffset=0  TranslationROffsetUnits=m  TranslationZOffset=0  TranslationZOffsetUnits=m  TranslationThetaOffset=0  TranslationThetaOffsetUnits=deg  RotationMethod=AlignedAxes  RotationAngleUnits=deg  RotationStandardAxis=+Z  RotationAngle=0.0  RotationArbitraryAxis=[0 0 1]  FollAlignAxisA=+Z  BaseAlignAxisA=+Y  FollAlignAxisB=+X  BaseAlignAxisB=+Z  RotationSequenceAxes=FollowerAxes  RotationSequence=XYX  RotationSequenceAngles=[0 0 0]  RotationSequenceAnglesUnits=deg  RotationMatrix=[1 0 0; 0 1 0; 0 0 1]
  Vertical Beam1 : $bdroot/Hollow Brick  width=beamWidth  depth=depth  length=vertBeamLength  thickness=beamThickness  rho=rho  color=beamColor
  Vertical Beam1 xForm : sm_lib/Frames and Transforms/Rigid Transform  TranslationMethod=Cartesian  TranslationStandardOffset=0  TranslationLengthUnit=m  TranslationStandardAxis=+Z  TranslationCartesianOffset=vertBeam1_offset  TranslationROffset=0  TranslationROffsetUnits=m  TranslationZOffset=0  TranslationZOffsetUnits=m  TranslationThetaOffset=0  TranslationThetaOffsetUnits=deg  RotationMethod=AlignedAxes  RotationAngleUnits=deg  RotationStandardAxis=+Z  RotationAngle=0.0  RotationArbitraryAxis=[0 0 1]  FollAlignAxisA=+Z  BaseAlignAxisA=+X  FollAlignAxisB=+X  BaseAlignAxisB=+Z  RotationSequenceAxes=FollowerAxes  RotationSequence=XYX  RotationSequenceAngles=[0 0 0]  RotationSequenceAnglesUnits=deg  RotationMatrix=[1 0 0; 0 1 0; 0 0 1]
  Vertical Beam2 : $bdroot/Hollow Brick  width=beamWidth  depth=depth  length=vertBeamLength  thickness=beamThickness  rho=rho  color=beamColor
  Vertical Beam2 xForm : sm_lib/Frames and Transforms/Rigid Transform  TranslationMethod=Cartesian  TranslationStandardOffset=0  TranslationLengthUnit=m  TranslationStandardAxis=+Z  TranslationCartesianOffset=vertBeam2_offset  TranslationROffset=0  TranslationROffsetUnits=m  TranslationZOffset=0  TranslationZOffsetUnits=m  TranslationThetaOffset=0  TranslationThetaOffsetUnits=deg  RotationMethod=AlignedAxes  RotationAngleUnits=deg  RotationStandardAxis=+Z  RotationAngle=0.0  RotationArbitraryAxis=[0 0 1]  FollAlignAxisA=+Z  BaseAlignAxisA=+X  FollAlignAxisB=+X  BaseAlignAxisB=+Z  RotationSequenceAxes=FollowerAxes  RotationSequence=XYX  RotationSequenceAngles=[0 0 0]  RotationSequenceAnglesUnits=deg  RotationMatrix=[1 0 0; 0 1 0; 0 0 1]
  B : PMIOPort  Side=Left
  T : PMIOPort  Port=2  Side=Right
  connections:
  Base xForm/LConn1 -- Far Frame xForm/LConn1 -- Top xForm/LConn1 -- Horizontal Beam/LConn1 -- Left Frame xForm/LConn1 -- Near Frame xForm/LConn1
  Base xForm/RConn1 -- B/RConn1
  Left Frame/LConn1 -- Left Frame xForm/RConn1
  Right Frame xForm/LConn1 -- Vertical Beam2 xForm/LConn1 -- Horizontal Beam/RConn1 -- Vertical Beam1 xForm/LConn1
  Right Frame xForm/RConn1 -- Right Frame/LConn1
  Top xForm/RConn1 -- T/RConn1
  Near Frame/LConn1 -- Near Frame xForm/RConn1
  Far Frame/LConn1 -- Far Frame xForm/RConn1
  Vertical Beam1 xForm/RConn1 -- Vertical Beam1/LConn1
  Vertical Beam2/LConn1 -- Vertical Beam2 xForm/RConn1

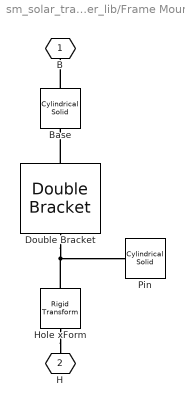
== system sm_solar_tracker_lib/Frame Mount ==
  Base : sm_lib/Body Elements/Cylindrical Solid  GraphicAmbientColor=[0.15 0.15 0.15 1.0]  BasedOnType=Density  CenterOfMass=[0 0 0]  CenterOfMassUnits=m  GraphicDiffuseColor=mountColor  CylinderLength=baseThickness  CylinderLengthUnits=m  CylinderRadius=baseRadius  CylinderRadiusUnits=m  Density=rho  DensityUnits=kg/m^3  DoExposeReferenceFrame=off  GraphicEmissiveColor=[0.0 0.0 0.0 1.0]  ExportEntireGeometry=off  SerializedFrames=<Frames><Frame><Id>Frame1</Id><Value><Name>T</Name><Origin><Source>GeometricFeature</Source><FeatureName>top surface</FeatureName></Origin><PrimaryAxis><DefinedDirection>+Z</DefinedDirection><Source>ReferenceFrame</Source><SourceDirection>+Z</SourceDirection><FeatureName></FeatureName></PrimaryAxis><SecondaryAxis><DefinedDirection>+X</DefinedDirection><Source>ReferenceFrame</Source><SourceDirection>+X</SourceDirection><FeatureName></FeatureName></SecondaryAxis></Value></Frame><Frame><Id>Frame2</Id><Value><Name>B</Name><Origin><Source>GeometricFeature</Source><FeatureName>bottom surface</FeatureName></Origin><PrimaryAxis><DefinedDirection>+Z</DefinedDirection><Source>ReferenceFrame</Source><SourceDirection>-Z</SourceDirection><FeatureName></FeatureName></PrimaryAxis><SecondaryAxis><DefinedDirection>+X</DefinedDirection><Source>ReferenceFrame</Source><SourceDirection>+Y</SourceDirection><FeatureName></FeatureName></SecondaryAxis></Value></Frame></Frames>  MarkerShape=Sphere  MarkerSize=10  GraphicType=FromGeometry  InertiaType=CalculateFromGeometry  Mass=1  MassUnits=kg  MomentsOfInertia=[1 1 1]  MomentsOfInertiaUnits=kg*m^2  GraphicOpacity=1.0  ProductsOfInertia=[1 1 1]  ProductsOfInertiaUnits=kg*m^2  GraphicShininess=75  GraphicSpecularColor=[0.5 0.5 0.5 1.0]  GraphicVisPropType=SimpleVisualProperties
  Double Bracket : $bdroot/Double Bracket  height=bracketWidth  width=bracketWidth  thickness=bracketThickness  offset=bracketOffset  holeOffset=holeOffset  holeRadius=holeRadius  rho=rho  color=mountColor
  Hole xForm : sm_lib/Frames and Transforms/Rigid Transform  TranslationMethod=None  TranslationStandardOffset=0  TranslationLengthUnit=m  TranslationStandardAxis=+Z  TranslationCartesianOffset=[0 0 0]  TranslationROffset=0  TranslationROffsetUnits=m  TranslationZOffset=0  TranslationZOffsetUnits=m  TranslationThetaOffset=0  TranslationThetaOffsetUnits=deg  RotationMethod=AlignedAxes  RotationAngleUnits=deg  RotationStandardAxis=+Z  RotationAngle=0.0  RotationArbitraryAxis=[0 0 1]  FollAlignAxisA=+Z  BaseAlignAxisA=+Z  FollAlignAxisB=+Y  BaseAlignAxisB=-Y  RotationSequenceAxes=FollowerAxes  RotationSequence=XYX  RotationSequenceAngles=[0 0 0]  RotationSequenceAnglesUnits=deg  RotationMatrix=[1 0 0; 0 1 0; 0 0 1]
  Pin : sm_lib/Body Elements/Cylindrical Solid  GraphicAmbientColor=[0.15 0.15 0.15 1.0]  BasedOnType=Density  CenterOfMass=[0 0 0]  CenterOfMassUnits=m  GraphicDiffuseColor=pinColor  CylinderLength=pinLength  CylinderLengthUnits=m  CylinderRadius=holeRadius  CylinderRadiusUnits=m  Density=rho  DensityUnits=kg/m^3  DoExposeReferenceFrame=on  GraphicEmissiveColor=[0.0 0.0 0.0 1.0]  ExportEntireGeometry=off  SerializedFrames=<Frames/>  MarkerShape=Sphere  MarkerSize=10  GraphicType=FromGeometry  InertiaType=CalculateFromGeometry  Mass=1  MassUnits=kg  MomentsOfInertia=[1 1 1]  MomentsOfInertiaUnits=kg*m^2  GraphicOpacity=1.0  ProductsOfInertia=[1 1 1]  ProductsOfInertiaUnits=kg*m^2  GraphicShininess=75  GraphicSpecularColor=[0.5 0.5 0.5 1.0]  GraphicVisPropType=SimpleVisualProperties
  B : PMIOPort  Side=Left
  H : PMIOPort  Port=2  Side=Right
  connections:
  Base/RConn1 -- B/RConn1
  Double Bracket/RConn1 -- Hole xForm/LConn1 -- Pin/RConn1
  Double Bracket/LConn1 -- Base/LConn1
  Hole xForm/RConn1 -- H/RConn1

== system sm_solar_tracker_lib/Hollow Brick ==
  Brick : sm_lib/Body Elements/Extruded Solid  GraphicAmbientColor=[0.15 0.15 0.15 1.0]  BasedOnType=Density  CenterOfMass=[0 0 0]  CenterOfMassUnits=m  GraphicDiffuseColor=color  ExportConvexHullGeometry=off  ExtrusionCrossSection=crossSection  ExtrusionCrossSectionUnits=m  Density=rho  DensityUnits=kg/m^3  DoExposeReferenceFrame=on  GraphicEmissiveColor=[0.0 0.0 0.0 1.0]  ExportEntireGeometry=off  ExtrusionLength=length  ExtrusionLengthUnits=m  ExtrusionType=General  SerializedFrames=<Frames/>  MarkerShape=Sphere  MarkerSize=10  GraphicType=FromGeometry  InertiaType=CalculateFromGeometry  Mass=1  MassUnits=kg  MomentsOfInertia=[1 1 1]  MomentsOfInertiaUnits=kg*m^2  PolygonNumSides=3  GraphicOpacity=1.0  PolygonOuterRadius=1  PolygonOuterRadiusUnits=m  ProductsOfInertia=[1 1 1]  ProductsOfInertiaUnits=kg*m^2  GraphicShininess=75  GraphicSpecularColor=[0.5 0.5 0.5 1.0]  GraphicVisPropType=SimpleVisualProperties
  Left xForm : sm_lib/Frames and Transforms/Rigid Transform  TranslationMethod=StandardAxis  TranslationStandardOffset=0.5*length  TranslationLengthUnit=m  TranslationStandardAxis=-Z  TranslationCartesianOffset=[0 0 0]  TranslationROffset=0  TranslationROffsetUnits=m  TranslationZOffset=0  TranslationZOffsetUnits=m  TranslationThetaOffset=0  TranslationThetaOffsetUnits=deg  RotationMethod=None  RotationAngleUnits=deg  RotationStandardAxis=+Z  RotationAngle=0.0  RotationArbitraryAxis=[0 0 1]  FollAlignAxisA=+X  BaseAlignAxisA=+Y  FollAlignAxisB=+Y  BaseAlignAxisB=+Z  RotationSequenceAxes=FollowerAxes  RotationSequence=XYX  RotationSequenceAngles=[0 0 0]  RotationSequenceAnglesUnits=deg  RotationMatrix=[1 0 0; 0 1 0; 0 0 1]
  Right xForm : sm_lib/Frames and Transforms/Rigid Transform  TranslationMethod=StandardAxis  TranslationStandardOffset=0.5*length  TranslationLengthUnit=m  TranslationStandardAxis=+Z  TranslationCartesianOffset=[0 0 0]  TranslationROffset=0  TranslationROffsetUnits=m  TranslationZOffset=0  TranslationZOffsetUnits=m  TranslationThetaOffset=0  TranslationThetaOffsetUnits=deg  RotationMethod=None  RotationAngleUnits=deg  RotationStandardAxis=+Z  RotationAngle=0.0  RotationArbitraryAxis=[0 0 1]  FollAlignAxisA=+X  BaseAlignAxisA=+Y  FollAlignAxisB=+Y  BaseAlignAxisB=+Z  RotationSequenceAxes=FollowerAxes  RotationSequence=XYX  RotationSequenceAngles=[0 0 0]  RotationSequenceAnglesUnits=deg  RotationMatrix=[1 0 0; 0 1 0; 0 0 1]
  L : PMIOPort  Side=Left
  R : PMIOPort  Port=2  Side=Right
  connections:
  Brick/RConn1 -- Right xForm/LConn1 -- Left xForm/LConn1
  Left xForm/RConn1 -- L/RConn1
  R/RConn1 -- Right xForm/RConn1

== system sm_solar_tracker_lib/Hollow Cylinder ==
  Cylinder : sm_lib/Body Elements/Revolved Solid  GraphicAmbientColor=[0.15 0.15 0.15 1.0]  BasedOnType=Density  CenterOfMass=[0 0 0]  CenterOfMassUnits=m  GraphicDiffuseColor=color  ExportConvexHullGeometry=off  Density=rho  DensityUnits=kg/m^3  DoExposeReferenceFrame=off  GraphicEmissiveColor=[0.0 0.0 0.0 1.0]  ExportEntireGeometry=off  SerializedFrames=<Frames><Frame><Id>Frame1</Id><Value><Name>L</Name><Origin><Source>GeometricFeature</Source><FeatureName>side surface 1</FeatureName></Origin><PrimaryAxis><DefinedDirection>+Z</DefinedDirection><Source>ReferenceFrame</Source><SourceDirection>+Z</SourceDirection><FeatureName></FeatureName></PrimaryAxis><SecondaryAxis><DefinedDirection>+X</DefinedDirection><Source>ReferenceFrame</Source><SourceDirection>+X</SourceDirection><FeatureName></FeatureName></SecondaryAxis></Value></Frame><Frame><Id>Frame2</Id><Value><Name>R</Name><Origin><Source>GeometricFeature</Source><FeatureName>side surface 3</FeatureName></Origin><PrimaryAxis><DefinedDirection>+Z</DefinedDirection><Source>ReferenceFrame</Source><SourceDirection>+Z</SourceDirection><FeatureName></FeatureName></PrimaryAxis><SecondaryAxis><DefinedDirection>+X</DefinedDirection><Source>ReferenceFrame</Source><SourceDirection>+X</SourceDirection><FeatureName></FeatureName></SecondaryAxis></Value></Frame></Frames>  MarkerShape=Sphere  MarkerSize=10  GraphicType=FromGeometry  InertiaType=CalculateFromGeometry  Mass=1  MassUnits=kg  MomentsOfInertia=[1 1 1]  MomentsOfInertiaUnits=kg*m^2  GraphicOpacity=1.0  ProductsOfInertia=[1 1 1]  ProductsOfInertiaUnits=kg*m^2  RevolutionCrossSection=crossSection  RevolutionCrossSectionUnits=m  RevolutionAngle=180  RevolutionAngleUnits=deg  RevolutionExtent=Full  GraphicShininess=75  GraphicSpecularColor=[0.5 0.5 0.5 1.0]  GraphicVisPropType=SimpleVisualProperties
  L : PMIOPort  Side=Left
  R : PMIOPort  Port=2  Side=Right
  connections:
  Cylinder/LConn1 -- L/RConn1
  R/RConn1 -- Cylinder/RConn1
